simulink model "control_sipro_wController"  (R2020b)
settings: Solver=VariableStepAuto  StartTime=0.0  StopTime=10.0  RelTol=1e-3
undefined symbols (not defined in the file): A, atilde, B, btilde, C, D, KD, KI, KP, ts
libraries: simulink x2
settings Model: Creator=Sampreet Sarkar  LastModifiedBy=yukisaito
settings DataIOCC: ReturnWorkspaceOutputs=off
settings DebuggingCC: ArithmeticOperatorsInVariantConditions=warning
settings SFSimCC: SimUseLocalCustomCode=off  CustomCodeUndefinedFunction=UseInterfaceOnly
settings RTWCC: RTWUseLocalCustomCode=off

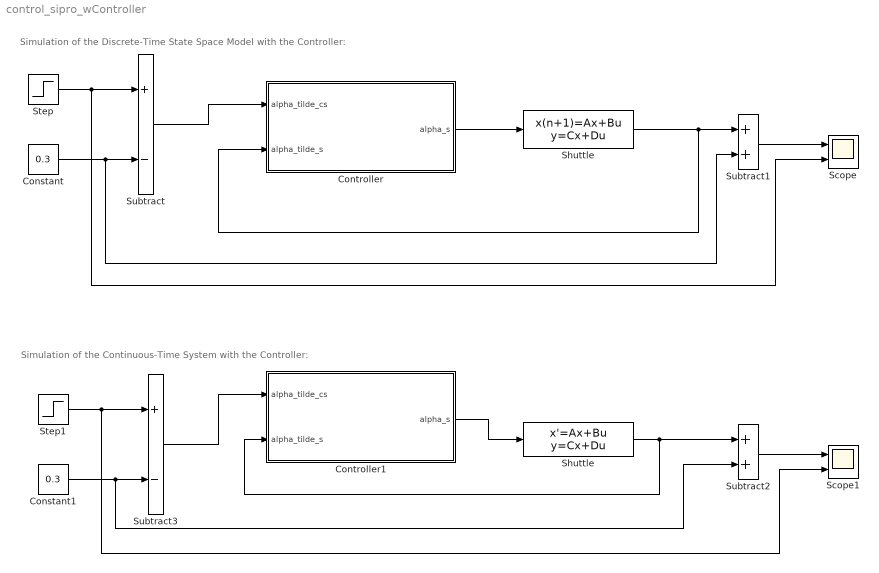
== system control_sipro_wController ==
  note: Simulation of the Continuous-Time System with the Controller:
  note: Simulation of the Discrete-Time State Space Model with the Controller:
  Constant : Constant  Value=0.3
  Constant1 : Constant  Value=0.3
  Controller : Subsystem
  Controller1 : Subsystem
  Scope : Scope  NumInputPorts=2
  Scope1 : Scope  NumInputPorts=2
  Shuttle : StateSpace  A=A  B=B  C=C  D=D  InitialCondition=0
  "Shuttle " : DiscreteStateSpace  A=atilde  B=btilde  C=C  D=D  SampleTime=ts
  Step : Step  Before=0.3  After=0.27  SampleTime=ts
  Step1 : Step  Before=0.3  After=0.27  SampleTime=ts
  Subtract : Sum  Inputs=+-
  Subtract1 : Sum
  Subtract2 : Sum
  Subtract3 : Sum  Inputs=+-
  wires:
  Controller/1(alpha_s) -> "Shuttle "/1
  Step/1 -> Scope/2, Subtract/1
  Constant/1 -> Subtract1/2, Subtract/2
  "Shuttle "/1 -> Controller/2(alpha_tilde_s), Subtract1/1
  Subtract/1 -> Controller/1(alpha_tilde_cs)
  Subtract1/1 -> Scope/1
  Shuttle/1 -> Controller1/2(alpha_tilde_s), Subtract2/1
  Subtract2/1 -> Scope1/1
  Step1/1 -> Scope1/2, Subtract3/1
  Constant1/1 -> Subtract2/2, Subtract3/2
  Subtract3/1 -> Controller1/1(alpha_tilde_cs)
  Controller1/1(alpha_s) -> Shuttle/1

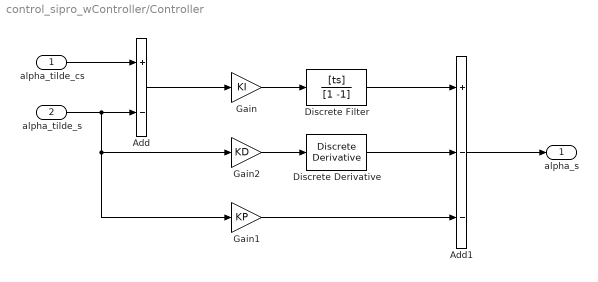
== system control_sipro_wController/Controller ==
  alpha_tilde_cs : Inport
  alpha_tilde_s : Inport  Port=2
  Add : Sum  Inputs=+-
  Add1 : Sum  Inputs=+--
  Discrete Derivative : simulink/Discrete/Discrete Derivative  gainval=1.0  ICPrevScaledInput=0.0  OutMin=[]  OutMax=[]  OutDataType=fixdt(1, 16)  OutScaling=2^-10  DoSatur=off
  Discrete Filter : DiscreteFilter  Numerator=[ts]  Denominator=[1 -1]
  Gain : Gain  Gain=KI
  Gain1 : Gain  Gain=KP
  Gain2 : Gain  Gain=KD
  alpha_s : Outport  VectorParamsAs1DForOutWhenUnconnected=off
  wires:
  Gain2/1 -> Discrete Derivative/1
  Discrete Filter/1 -> Add1/1
  Add/1 -> Gain/1
  Gain/1 -> Discrete Filter/1
  alpha_tilde_s/1 -> Gain1/1, Gain2/1, Add/2
  Discrete Derivative/1 -> Add1/2
  alpha_tilde_cs/1 -> Add/1
  Gain1/1 -> Add1/3
  Add1/1 -> alpha_s/1

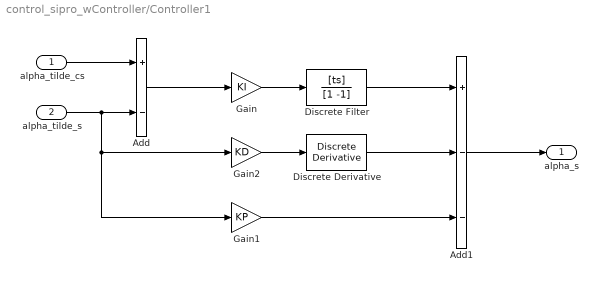
== system control_sipro_wController/Controller1 ==
  alpha_tilde_cs : Inport
  alpha_tilde_s : Inport  Port=2
  Add : Sum  Inputs=+-
  Add1 : Sum  Inputs=+--
  Discrete Derivative : simulink/Discrete/Discrete Derivative  gainval=1.0  ICPrevScaledInput=0.0  OutMin=[]  OutMax=[]  OutDataType=fixdt(1, 16)  OutScaling=2^-10  DoSatur=off
  Discrete Filter : DiscreteFilter  Numerator=[ts]  Denominator=[1 -1]
  Gain : Gain  Gain=KI
  Gain1 : Gain  Gain=KP
  Gain2 : Gain  Gain=KD
  alpha_s : Outport  VectorParamsAs1DForOutWhenUnconnected=off
  wires:
  Gain2/1 -> Discrete Derivative/1
  Discrete Filter/1 -> Add1/1
  Add/1 -> Gain/1
  Gain/1 -> Discrete Filter/1
  alpha_tilde_s/1 -> Gain1/1, Gain2/1, Add/2
  Discrete Derivative/1 -> Add1/2
  alpha_tilde_cs/1 -> Add/1
  Gain1/1 -> Add1/3
  Add1/1 -> alpha_s/1
